simulink model "zuni"  (R2019b)
settings: Solver=FixedStepAuto  StartTime=0.0  StopTime=20.0  RelTol=1e-3
settings Model: Creator=eden  LastModifiedBy=eden
settings SolverCC: InitialStep=0.1

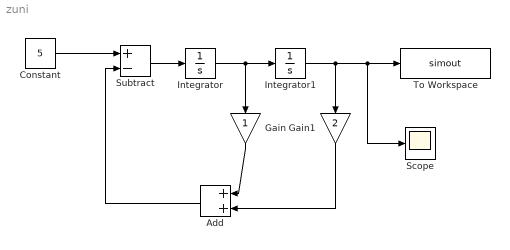
== system zuni ==
  Add : Sum
  Constant : Constant  Value=5
  Gain : Gain
  Gain1 : Gain  Gain=2
  Integrator : Integrator
  Integrator1 : Integrator
  Scope : Scope
  Subtract : Sum  Inputs=+-
  To Workspace : ToWorkspace  VariableName=simout  SaveFormat=Timeseries  SampleTime=-1
  wires:
  Constant/1 -> Subtract/1
  Add/1 -> Subtract/2
  Subtract/1 -> Integrator/1
  Integrator/1 -> Gain/1, Integrator1/1
  Gain/1 -> Add/1
  Gain1/1 -> Add/2
  Integrator1/1 -> Scope/1, To Workspace/1, Gain1/1
